simulink model "simulink_tarefa3"  (R2022b)
settings: Solver=VariableStepAuto  StartTime=0.0  StopTime=15  RelTol=1e-3
settings Model: Creator=hugo_  LastModifiedBy=hugo_

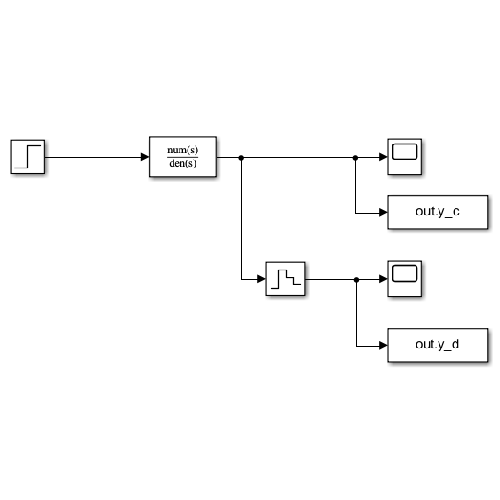
[thumbnail: Simulink's stored preview of the top-level diagram]
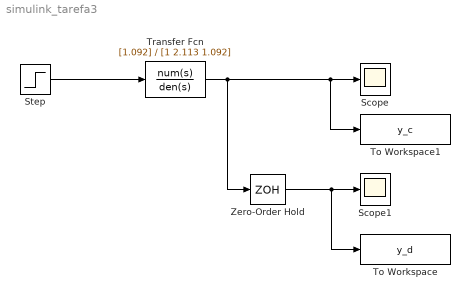
== system simulink_tarefa3 ==
  Scope : Scope
  Scope1 : Scope
  Step : Step  Time=0  After=1.25  SampleTime=0
  To Workspace : ToWorkspace  VariableName=y_d  SaveFormat=Timeseries  SampleTime=-1
  To Workspace1 : ToWorkspace  VariableName=y_c  SaveFormat=Timeseries  SampleTime=-1
  Transfer Fcn : TransferFcn  Numerator=[1.092]  Denominator=[1 2.113 1.092]
  Zero-Order Hold : ZeroOrderHold  SampleTime=0.951
  wires:
  Step/1 -> Transfer Fcn/1
  Transfer Fcn/1 -> Zero-Order Hold/1, To Workspace1/1, Scope/1
  Zero-Order Hold/1 -> To Workspace/1, Scope1/1
